simulink model "fourBebop_circle"  (R2017b)
settings: Solver=FixedStepAuto  StartTime=0.0  StopTime=inf  FixedStep=sampleTime  RelTol=1e-3  EnableMultiTasking=on
undefined symbols (not defined in the file or in its folder): Angular, Linear, R
libraries: simulink x20, robotlib x20
(part 2 of 2)

== matlab function fourBebop_circle/Baseline Controller4/MATLAB Function ==
  data: u input; y output; a input
function y = fcn(u,a)
y = satgd(u,a);

== matlab function fourBebop_circle/Baseline Controller4/Position controller/Coordinate trnasformation from inertial frame to body frame  ==
  data: Vec_i input; Vec_xy output; psi input
function Vec_xy  = fcn(Vec_i , psi)
%#codegen
T = [cos(psi) sin(psi) ; -sin(psi) cos(psi)] ; 
Vec_xy = T*Vec_i(1:2,1);

== matlab function fourBebop_circle/MATLAB Function3 ==
  data: u input; y output; lostsigalcount input
function y = fcn(u,lostsigalcount)


if  -0.00001<u & u<0.00001
    lostsigalcount = lostsigalcount +1;
else
    lostsigalcount = 0;
end

if lostsigalcount>=3
  y=0;
else
  y=1;
end

== matlab function fourBebop_circle/ang4/  ==
  data: ang_x output; X input; ang_y output; Y input; Z input; ang_z output
function [ang_x, ang_y, ang_z] = angle_tf(X, Y, Z)
ang_x =  X*pi/180;
ang_y =  -Y*pi/180;
ang_z =  -Z*pi/180;

== matlab function fourBebop_circle/pos4/  ==
  data: vps_x output; vps_X input; vps_y output; vps_Y input; vps_Z input; vps_z output
function [vps_x, vps_y, vps_z] = xyz_offset(vps_X, vps_Y, vps_Z)
% x =  vps_X + offset_X;
% y =  -vps_Y+offset_Y;
% z =  vps_Z+offset_Z;
temp=[vps_X;vps_Y;vps_Z];
vps_x=temp(1);
vps_y=temp(2);
vps_z=temp(3);

== matlab function fourBebop_circle/vel3/ 2 ==
  data: vps_vx output; vps_X input; vps_vy output; vps_Y input; vps_Z input; vps_vz output
function [vps_vx, vps_vy, vps_vz] = vxyz_offset(vps_X, vps_Y, vps_Z)
% x =  vps_X + offset_X;
% y =  -vps_Y+offset_Y;
% z =  vps_Z+offset_Z;
temp=[vps_X;vps_Y;vps_Z];
vps_vx=temp(1);
vps_vy=temp(2);
vps_vz=temp(3);
